simulink library "LearningLib"  (Simulink 7.7)
settings: Solver=ode45  SolverMode=SingleTasking  StartTime=0.0  StopTime=10.0  RelTol=1e-3
undefined symbols (not defined in the file or in its folder): magnitude
settings Model: Creator=jpalma  LastModifiedBy=jpalma

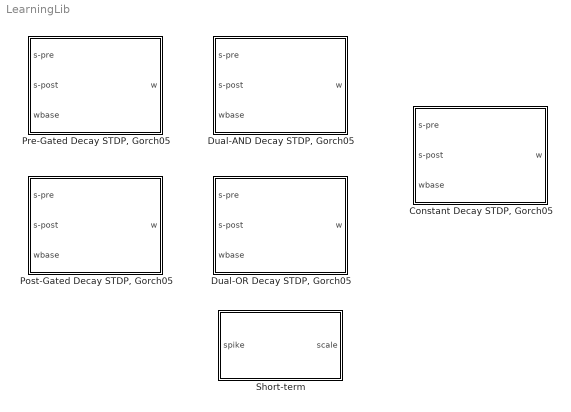
== system LearningLib ==
  "Constant Decay STDP, Gorch05" : Subsystem  mask{lamb=1, w_0=0.5, w_range=2, dec=0.04}
      mask prompts: lamb "Learning Rate, lambda"; w_0 "Weight equilibrium point, w_0"; w_range "Weight Range, w_max - w_min"; dec "decay constant"
      mask Display: image(imread('../Libs/icons/STDP.JPG'),'center');
  "Dual-AND Decay STDP, Gorch05" : Subsystem  mask{lamb=1, w_0=0.5, w_range=2, c=1}
      mask prompts: lamb "Learning Rate, lambda"; w_0 "Weight equilibrium point, w_0"; w_range "Weight Range, w_max - w_min"; c "c gain"
      mask Display: image(imread('../Libs/icons/STDP.JPG'),'center');
  "Dual-OR Decay STDP, Gorch05" : Subsystem  mask{lamb=1, w_0=0.5, w_range=2, a=2, b=2}
      mask prompts: lamb "Learning Rate, lambda"; w_0 "Weight equilibrium point, w_0"; w_range "Weight Range, w_max - w_min"; a "a gain"; b "b gain"
      mask Display: image(imread('../Libs/icons/STDP.JPG'),'center');
  "Post-Gated Decay STDP, Gorch05" : Subsystem  mask{lamb=1, w_0=0.5, w_range=2, b=2}
      mask prompts: lamb "Learning Rate, lambda"; w_0 "Weight equilibrium point, w_0"; w_range "Weight Range, w_max - w_min"; b "b gain"
      mask Display: image(imread('../Libs/icons/STDP.JPG'),'center');
  "Pre-Gated Decay STDP, Gorch05" : Subsystem  mask{lamb=1, w_0=0.5, w_range=2, a=2}
      mask prompts: lamb "Learning Rate, lambda"; w_0 "Weight equilibrium point, w_0"; w_range "Weight Range, w_max - w_min"; a "a gain"
      mask Display: image(imread('../Libs/icons/STDP.JPG'),'center');
  Short-term : Subsystem  mask{tau=60, p_gain=6}
      mask prompts: tau "Time Constant, tau"; p_gain "Gain effect, p_gain"
      mask Display: image(imread('../Libs/icons/ShortT.JPG'),'center');

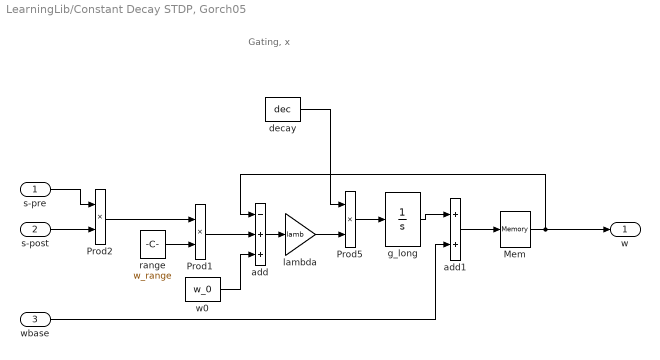
== system LearningLib/Constant Decay STDP, Gorch05 ==
  note: Gating, x
  s-pre : Inport
  s-post : Inport  Port=2
  wbase : Inport  Port=3
  Mem : Memory
  Prod1 : Product  RndMeth=Zero
  Prod2 : Product  RndMeth=Zero
  Prod5 : Product  RndMeth=Zero
  add : Sum  Inputs=-++
  add1 : Sum
  decay : Constant  Value=dec
  g_long : Integrator  ZeroCross=off
  lambda : Gain  Gain=lamb
  range : Constant  Value=w_range
  w0 : Constant  Value=w_0
  w : Outport
  wires:
  Mem/1 -> add/1, w/1
  add/1 -> lambda/1
  range/1 -> Prod1/2
  Prod2/1 -> Prod1/1
  Prod1/1 -> add/2
  Prod5/1 -> g_long/1
  lambda/1 -> Prod5/2
  s-post/1 -> Prod2/2
  s-pre/1 -> Prod2/1
  w0/1 -> add/3
  g_long/1 -> add1/1
  wbase/1 -> add1/2
  add1/1 -> Mem/1
  decay/1 -> Prod5/1

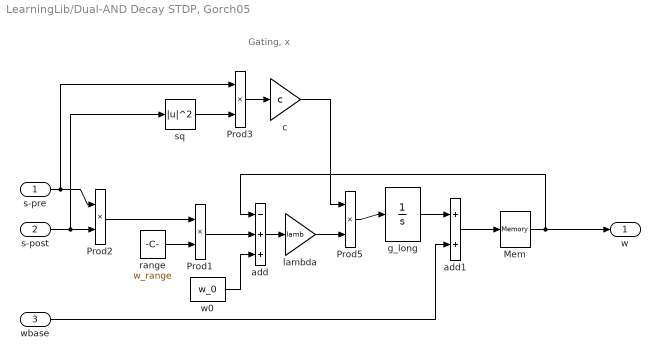
== system LearningLib/Dual-AND Decay STDP, Gorch05 ==
  note: Gating, x
  s-pre : Inport
  s-post : Inport  Port=2
  wbase : Inport  Port=3
  Mem : Memory
  Prod{1..3,5} (4 alike) : Product  RndMeth=Zero
  add : Sum  Inputs=-++
  add1 : Sum
  c : Gain  Gain=c
  g_long : Integrator  ZeroCross=off
  lambda : Gain  Gain=lamb
  range : Constant  Value=w_range
  sq : Math  Operator=magnitude^2  SaturateOnIntegerOverflow=on
  w0 : Constant  Value=w_0
  w : Outport
  wires:
  Mem/1 -> add/1, w/1
  add/1 -> lambda/1
  range/1 -> Prod1/2
  Prod2/1 -> Prod1/1
  Prod1/1 -> add/2
  Prod5/1 -> g_long/1
  lambda/1 -> Prod5/2
  s-post/1 -> Prod2/2, sq/1
  s-pre/1 -> Prod2/1, Prod3/1
  w0/1 -> add/3
  g_long/1 -> add1/1
  wbase/1 -> add1/2
  add1/1 -> Mem/1
  sq/1 -> Prod3/2
  Prod3/1 -> c/1
  c/1 -> Prod5/1

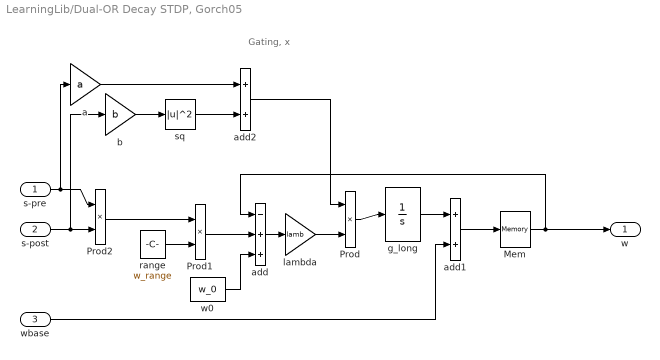
== system LearningLib/Dual-OR Decay STDP, Gorch05 ==
  note: Gating, x
  s-pre : Inport
  s-post : Inport  Port=2
  wbase : Inport  Port=3
  Mem : Memory
  Prod : Product  RndMeth=Zero
  Prod1 : Product  RndMeth=Zero
  Prod2 : Product  RndMeth=Zero
  a : Gain  Gain=a
  add : Sum  Inputs=-++
  add1 : Sum
  add2 : Sum
  b : Gain  Gain=b
  g_long : Integrator  ZeroCross=off
  lambda : Gain  Gain=lamb
  range : Constant  Value=w_range
  sq : Math  Operator=magnitude^2  SaturateOnIntegerOverflow=on
  w0 : Constant  Value=w_0
  w : Outport
  wires:
  sq/1 -> add2/2
  add1/1 -> Mem/1
  wbase/1 -> add1/2
  g_long/1 -> add1/1
  w0/1 -> add/3
  s-pre/1 -> Prod2/1, a/1
  s-post/1 -> Prod2/2, b/1
  lambda/1 -> Prod/2
  Prod/1 -> g_long/1
  Prod1/1 -> add/2
  Prod2/1 -> Prod1/1
  range/1 -> Prod1/2
  add/1 -> lambda/1
  Mem/1 -> w/1, add/1
  a/1 -> add2/1
  b/1 -> sq/1
  add2/1 -> Prod/1

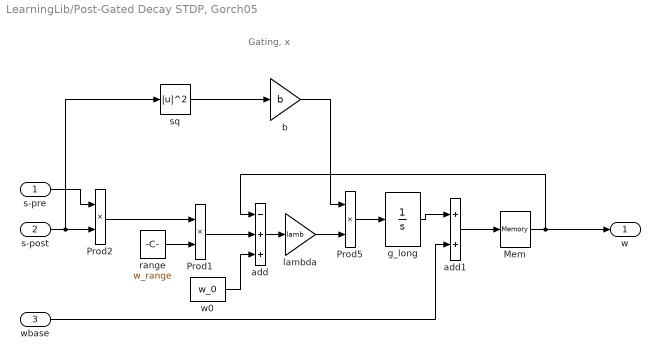
== system LearningLib/Post-Gated Decay STDP, Gorch05 ==
  note: Gating, x
  s-pre : Inport
  s-post : Inport  Port=2
  wbase : Inport  Port=3
  Mem : Memory
  Prod1 : Product  RndMeth=Zero
  Prod2 : Product  RndMeth=Zero
  Prod5 : Product  RndMeth=Zero
  add : Sum  Inputs=-++
  add1 : Sum
  b : Gain  Gain=b
  g_long : Integrator  ZeroCross=off
  lambda : Gain  Gain=lamb
  range : Constant  Value=w_range
  sq : Math  Operator=magnitude^2  SaturateOnIntegerOverflow=on
  w0 : Constant  Value=w_0
  w : Outport
  wires:
  Mem/1 -> add/1, w/1
  add/1 -> lambda/1
  range/1 -> Prod1/2
  Prod2/1 -> Prod1/1
  Prod1/1 -> add/2
  Prod5/1 -> g_long/1
  lambda/1 -> Prod5/2
  s-post/1 -> Prod2/2, sq/1
  s-pre/1 -> Prod2/1
  w0/1 -> add/3
  g_long/1 -> add1/1
  wbase/1 -> add1/2
  add1/1 -> Mem/1
  b/1 -> Prod5/1
  sq/1 -> b/1

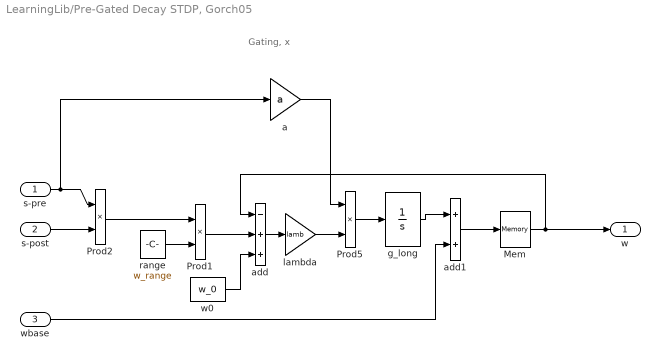
== system LearningLib/Pre-Gated Decay STDP, Gorch05 ==
  note: Gating, x
  s-pre : Inport
  s-post : Inport  Port=2
  wbase : Inport  Port=3
  Mem : Memory
  Prod1 : Product  RndMeth=Zero
  Prod2 : Product  RndMeth=Zero
  Prod5 : Product  RndMeth=Zero
  a : Gain  Gain=a
  add : Sum  Inputs=-++
  add1 : Sum
  g_long : Integrator  ZeroCross=off
  lambda : Gain  Gain=lamb
  range : Constant  Value=w_range
  w0 : Constant  Value=w_0
  w : Outport
  wires:
  a/1 -> Prod5/1
  add1/1 -> Mem/1
  wbase/1 -> add1/2
  g_long/1 -> add1/1
  w0/1 -> add/3
  s-pre/1 -> Prod2/1, a/1
  s-post/1 -> Prod2/2
  lambda/1 -> Prod5/2
  Prod5/1 -> g_long/1
  Prod1/1 -> add/2
  Prod2/1 -> Prod1/1
  range/1 -> Prod1/2
  add/1 -> lambda/1
  Mem/1 -> w/1, add/1

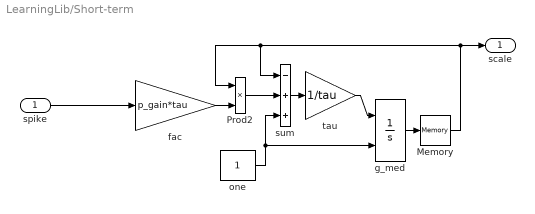
== system LearningLib/Short-term ==
  spike : Inport
  Memory : Memory
  Prod2 : Product  RndMeth=Zero
  fac : Gain  Gain=p_gain*tau
  g_med : Integrator  InitialConditionSource=external  ZeroCross=off
  one : Constant
  sum : Sum  Inputs=-++
  tau : Gain  Gain=1/tau
  scale : Outport
  wires:
  g_med/1 -> Memory/1
  Memory/1 -> sum/1, Prod2/1, scale/1
  fac/1 -> Prod2/2
  Prod2/1 -> sum/2
  sum/1 -> tau/1
  tau/1 -> g_med/1
  spike/1 -> fac/1
  one/1 -> sum/3, g_med/2
